simulink model "m13solm3"  (Simulink 8.9)
settings: Solver=ode4  StartTime=0.1  StopTime=1000  RelTol=1e-3  EnableMultiTasking=on
undefined symbols (not defined in the file): nmax, nmin, seed, tc
settings Model: Creator=Esben  LastModifiedBy=Roberto
settings DataIOCC: SignalLoggingSaveFormat=Dataset
settings OptimizationCC: ExpressionDepthLimit=2147483647
settings DebuggingCC: SolverPrmCheckMsg=warning

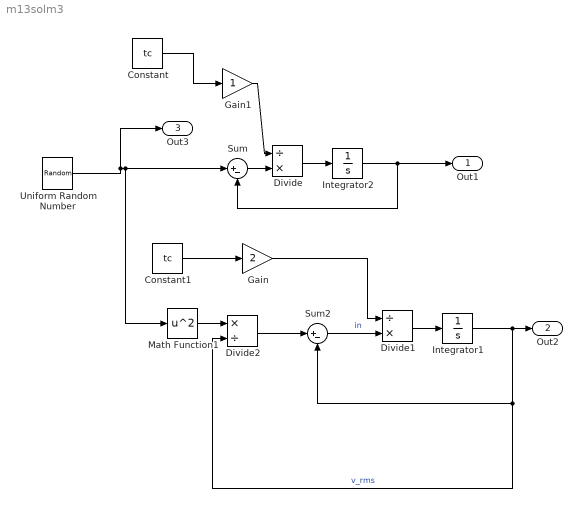
== system m13solm3 ==
  Constant : Constant  Value=tc
  Constant1 : Constant  Value=tc
  Divide : Product  Inputs=/*
  Divide1 : Product  Inputs=/*
  Divide2 : Product  Inputs=*/
  Gain : Gain  Gain=2
  Gain1 : Gain
  Integrator1 : Integrator  InitialCondition=0.001
  Integrator2 : Integrator  InitialCondition=0.0001
  Math Function1 : Math  Operator=square  SaturateOnIntegerOverflow=on
  Sum : Sum  Inputs=|+-
  Sum2 : Sum  Inputs=|+-
  Uniform Random Number : UniformRandomNumber  Minimum=nmin  Maximum=nmax  Seed=seed  SampleTime=1
  Out1 : Outport
  Out2 : Outport  Port=2
  Out3 : Outport  Port=3
  wires:
  Sum/1 -> Divide/2
  Divide/1 -> Integrator2/1
  Integrator2/1 -> Sum/2, Out1/1
  Divide1/1 -> Integrator1/1
  Integrator1/1 -> Sum2/2, Divide2/2, Out2/1  "v_rms"
  Gain/1 -> Divide1/1
  Sum2/1 -> Divide1/2  "in"
  Divide2/1 -> Sum2/1
  Math Function1/1 -> Divide2/1
  Gain1/1 -> Divide/1
  Uniform Random Number/1 -> Math Function1/1, Sum/1, Out3/1
  Constant/1 -> Gain1/1
  Constant1/1 -> Gain/1
